simulink model "power2"  (R2020b)
settings: Solver=VariableStepAuto  StartTime=0.0  StopTime=0.2  RelTol=1e-3
libraries: powerlib x39
settings Model: Creator=dhan  LastModifiedBy=dhan

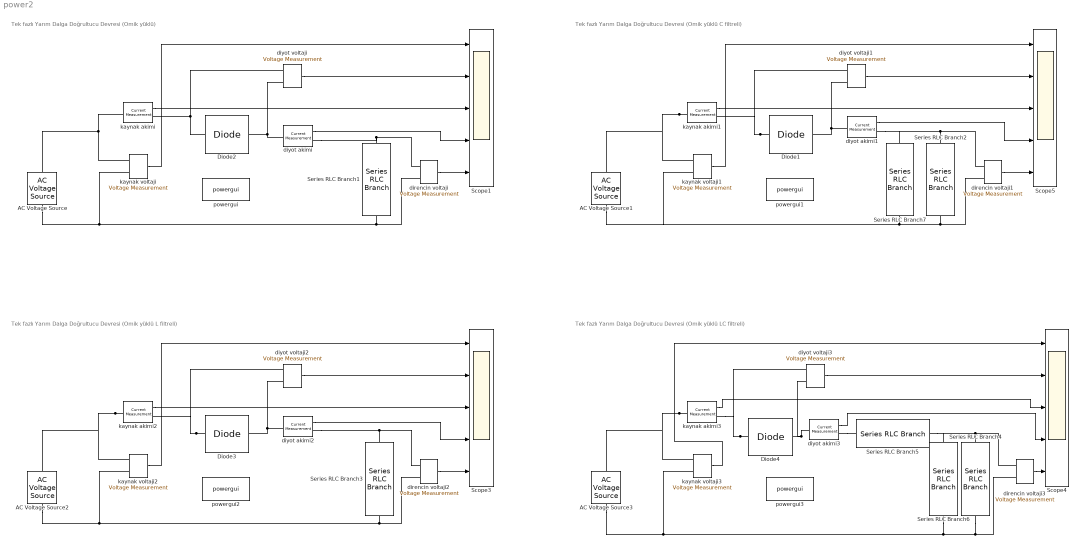
== system power2 ==
  note: Tek fazlı Yarım Dalga Doğrultucu Devresi (Omik yüklü)
  note: Tek fazlı Yarım Dalga Doğrultucu Devresi (Omik yüklü C filtreli)
  note: Tek fazlı Yarım Dalga Doğrultucu Devresi (Omik yüklü L filtreli)
  note: Tek fazlı Yarım Dalga Doğrultucu Devresi (Omik yüklü LC filtreli)
  AC Voltage Source{,1..3} (4 alike) : powerlib/Electrical Sources/AC Voltage Source  Amplitude=50  Phase=0  Frequency=50  SampleTime=0  Measurements=None  BusType=swing  Pref=10e3  Qref=0  Qmin=-inf  Qmax=+inf
  Diode{1..4} (4 alike) : powerlib/Power Electronics/Diode  Ron=0.001  Lon=0  Vf=0.8  IC=0  UseSnubber=0  Rs=500  Cs=250e-9  Measurements=off
  Scope{1,3..5} (4 alike) : Scope  NumInputPorts=5
  Series RLC Branch1 : powerlib/Elements/Series RLC Branch  LConnTagsString=__new0  RConnTagsString=__new0  BranchType=R  Resistance=20  Inductance=0  SetiL0=off  InitialCurrent=0  Capacitance=100*10^-6  Setx0=off  InitialVoltage=0  Measurements=None
  Series RLC Branch2 : powerlib/Elements/Series RLC Branch  LConnTagsString=__new0  RConnTagsString=__new0  BranchType=R  Resistance=20  Inductance=0  SetiL0=off  InitialCurrent=0  Capacitance=100*10^-6  Setx0=off  InitialVoltage=0  Measurements=None
  Series RLC Branch3 : powerlib/Elements/Series RLC Branch  LConnTagsString=__new0  RConnTagsString=__new0  BranchType=RL  Resistance=20  Inductance=27*10^-3  SetiL0=off  InitialCurrent=0  Capacitance=100*10^-6  Setx0=off  InitialVoltage=0  Measurements=None
  Series RLC Branch4 : powerlib/Elements/Series RLC Branch  LConnTagsString=__new0  RConnTagsString=__new0  BranchType=R  Resistance=20  Inductance=0  SetiL0=off  InitialCurrent=0  Capacitance=100*10^-6  Setx0=off  InitialVoltage=0  Measurements=None
  Series RLC Branch5 : powerlib/Elements/Series RLC Branch  LConnTagsString=__new0  RConnTagsString=__new0  BranchType=L  Resistance=20  Inductance=27*10^-3  SetiL0=off  InitialCurrent=0  Capacitance=100*10^-6  Setx0=off  InitialVoltage=0  Measurements=None
  Series RLC Branch6 : powerlib/Elements/Series RLC Branch  LConnTagsString=__new0  RConnTagsString=__new0  BranchType=C  Resistance=20  Inductance=0  SetiL0=off  InitialCurrent=0  Capacitance=100*10^-6  Setx0=off  InitialVoltage=0  Measurements=None
  Series RLC Branch7 : powerlib/Elements/Series RLC Branch  LConnTagsString=__new0  RConnTagsString=__new0  BranchType=C  Resistance=20  Inductance=0  SetiL0=off  InitialCurrent=0  Capacitance=100*10^-6  Setx0=off  InitialVoltage=0  Measurements=None
  direncin voltaji{,1..3} (4 alike) : powerlib/Measurements/Voltage Measurement  PhasorSimulation=off  OutputType=Complex  PSBequivalent=0
  diyot akimi{,1..3} (4 alike) : powerlib/Measurements/Current Measurement  PhasorSimulation=off  OutputType=Complex  PSBequivalent=0
  diyot voltaji{,1..3} (4 alike) : powerlib/Measurements/Voltage Measurement  PhasorSimulation=off  OutputType=Complex  PSBequivalent=0
  kaynak akimi{,1..3} (4 alike) : powerlib/Measurements/Current Measurement  PhasorSimulation=off  OutputType=Complex  PSBequivalent=0
  kaynak voltaji{,1..3} (4 alike) : powerlib/Measurements/Voltage Measurement  PhasorSimulation=off  OutputType=Complex  PSBequivalent=0
  powergui{,1..3} (4 alike) : powerlib/powergui  Priority=1  SimulationMode=Discrete  SampleTime=50e-6  frequency=60  Iterations=50  frequencyindice=50  Pbase=100e6  ErrMax=1e-4  UnitsV=kV  UnitsW=MW  buscounter=0  FunctionMessages=off  echomessages=off  EnableUseOfTLC=off  CurrentSourceSwitches=off  DisableSnubberDevices=off  DisableRonSwitches=off  DisableVfSwitches=off  DisplayEquations=off  AutomaticDiscreteSolvers=off  SolverType=Tustin/Backward Euler (TBE)  Interpol=off  ExternalGateDelay=off  methode=off  Ts=100  x0status=blocks  SPID=on  SwTol=0  HookPort=off  NonlinearTolerance=1e-4  nMaxIteration=100  ContinueOnMaxIteration=off  RestoreLinks=warning  ResistiveCurrentMeasurement=off  Frange=[0:2:500]  Ylog=off  Xlog=on  ShowGrid=off  save=off  variable=ZData  structure=0  ZoomFFT=off  StartTime=0.0  cycles=1  DisplayStyle=1  fundamental=60  FreqAxis=off  MaxFrequency=1000  frequencyindicesteady=1  RmsSteady=1  display=off
  wires:
  kaynak akimi/1 -> Scope1/3
  diyot voltaji/1 -> Scope1/2
  kaynak voltaji/1 -> Scope1/1
  diyot akimi/1 -> Scope1/4
  direncin voltaji/1 -> Scope1/5
  kaynak voltaji1/1 -> Scope5/1
  direncin voltaji1/1 -> Scope5/5
  kaynak akimi1/1 -> Scope5/3
  diyot voltaji1/1 -> Scope5/2
  diyot akimi1/1 -> Scope5/4
  kaynak akimi2/1 -> Scope3/3
  direncin voltaji2/1 -> Scope3/5
  kaynak voltaji2/1 -> Scope3/1
  diyot voltaji2/1 -> Scope3/2
  diyot akimi2/1 -> Scope3/4
  kaynak akimi3/1 -> Scope4/3
  direncin voltaji3/1 -> Scope4/5
  kaynak voltaji3/1 -> Scope4/1
  diyot voltaji3/1 -> Scope4/2
  diyot akimi3/1 -> Scope4/4
  connections:
  AC Voltage Source/RConn1 -- kaynak voltaji/LConn1 -- kaynak akimi/LConn1
  kaynak akimi/RConn1 -- diyot voltaji/LConn1 -- Diode2/LConn1
  diyot akimi/LConn1 -- diyot voltaji/LConn2 -- Diode2/RConn1
  diyot akimi/RConn1 -- Series RLC Branch1/LConn1 -- direncin voltaji/LConn1
  AC Voltage Source/LConn1 -- kaynak voltaji/LConn2 -- direncin voltaji/LConn2 -- Series RLC Branch1/RConn1
  direncin voltaji1/LConn1 -- Series RLC Branch2/LConn1 -- Series RLC Branch7/LConn1 -- diyot akimi1/RConn1
  diyot voltaji1/LConn2 -- Diode1/RConn1 -- diyot akimi1/LConn1
  kaynak akimi1/LConn1 -- AC Voltage Source1/RConn1 -- kaynak voltaji1/LConn1
  Diode1/LConn1 -- diyot voltaji1/LConn1 -- kaynak akimi1/RConn1
  Series RLC Branch2/RConn1 -- Series RLC Branch7/RConn1 -- AC Voltage Source1/LConn1 -- kaynak voltaji1/LConn2 -- direncin voltaji1/LConn2
  diyot voltaji2/LConn2 -- Diode3/RConn1 -- diyot akimi2/LConn1
  kaynak akimi2/LConn1 -- AC Voltage Source2/RConn1 -- kaynak voltaji2/LConn1
  kaynak voltaji2/LConn2 -- AC Voltage Source2/LConn1 -- Series RLC Branch3/LConn1 -- direncin voltaji2/LConn2
  diyot akimi2/RConn1 -- direncin voltaji2/LConn1 -- Series RLC Branch3/RConn1
  Diode3/LConn1 -- diyot voltaji2/LConn1 -- kaynak akimi2/RConn1
  diyot voltaji3/LConn2 -- diyot akimi3/LConn1 -- Diode4/RConn1
  kaynak akimi3/LConn1 -- AC Voltage Source3/RConn1 -- kaynak voltaji3/LConn1
  kaynak voltaji3/LConn2 -- AC Voltage Source3/LConn1 -- Series RLC Branch6/RConn1 -- Series RLC Branch4/RConn1 -- direncin voltaji3/LConn2
  direncin voltaji3/LConn1 -- Series RLC Branch5/LConn1 -- Series RLC Branch6/LConn1 -- Series RLC Branch4/LConn1
  Diode4/LConn1 -- diyot voltaji3/LConn1 -- kaynak akimi3/RConn1
  diyot akimi3/RConn1 -- Series RLC Branch5/RConn1
